simulink model "PackAndSend"  (R2016b)
settings: Solver=FixedStepDiscrete  StartTime=0.0  StopTime=inf  FixedStep=sCoreParams.core.stepPeriod  RelTol=1e-3  EnableMultiTasking=on
values from neighbouring files (symbols this model uses):
  sCoreParams = InitCoreParams    [ClosedLoopStimConsole.m]    (also in CompileModelComplete.m; NeuroModConsole.m)
libraries: simulink x2, xpclib x2
settings Model: Creator=User  LastModifiedBy=rzelmann
settings SolverCC: EnableConcurrentExecution=on
settings DataIOCC: SaveFormat=Array  SaveOutput=off  SignalLogging=off  DSMLogging=off  SaveTime=off
settings OptimizationCC: BlockReduction=off  DefaultParameterBehavior=Inlined  OptimizeBlockIOStorage=off  BufferReuse=off  GlobalBufferReuse=off  ExpressionFolding=off  LocalBlockOutputs=off
settings DebuggingCC: UnderspecifiedInitializationDetection=Classic  MergeDetectMultiDrivingBlocksExec=none  SolverPrmCheckMsg=warning  StateNameClashWarn=warning  SFUnexpectedBacktrackingDiag=warning  SFNoUnconditionalDefaultTransitionDiag=warning  SFExecutionAtInitializationDiag=none
settings HardwareCC: ProdBitPerPointer=32  ProdBitPerSizeT=32  ProdBitPerPtrDiffT=32  ProdLargestAtomicFloat=None  ProdWordSize=32  ProdLongLongMode=on  ProdHWDeviceType=Generic->32-bit x86 compatible
settings ModelReferenceCC: ModelReferenceNumInstancesAllowed=Single  PropagateSignalLabelsOutOfModel=off
settings RTWCC: SystemTargetFile=slrt.tlc  TemplateMakefile=slrt_default_tmf  Description=Simulink Real-Time  RTWCompilerOptimization=on
settings SimulinkRealTimeCC: xPCisModelTimeout=off
settings ConfigComp: CovMetricSettings=dw  CovHtmlReporting=on  CovSaveCumulativeToWorkspaceVar=on  CovSaveSingleToWorkspaceVar=on  CovExternalEMLEnable=off

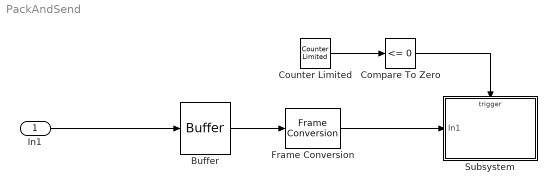
== system PackAndSend ==
  In1 : Inport  PortDimensions=[1 sCoreParams.write.maxSignalsPerStep]  SampleTime=sCoreParams.core.stepPeriod  Interpolate=off
  Buffer : Buffer  N=sCoreParams.write.broadcastSamp  V=sCoreParams.write.broadcastSamp-1  TreatMby1Signals=One channel
  Compare To Zero : simulink/Logic and Bit Operations/Compare To Zero  relop=<=  OutDataTypeStr=boolean
  Counter Limited : simulink/Sources/Counter Limited  uplimit=sCoreParams.write.broadcastSamp-1  tsamp=-1
  Frame Conversion : FrameConversion  InheritSamplingMode=off  OutFrame=Sample-based
  Subsystem : Subsystem
  wires:
  Buffer/1 -> Frame Conversion/1
  Counter Limited/1 -> Compare To Zero/1
  Compare To Zero/1 -> Subsystem/Trigger
  Frame Conversion/1 -> Subsystem/1(In1)
  In1/1 -> Buffer/1

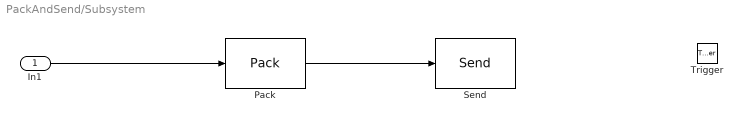
== system PackAndSend/Subsystem ==
  In1 : Inport
  Trigger : TriggerPort  VariantControl=Variant  PortDimensions=1
  Pack : xpclib/UDP/Pack  datatypes={'double'}  byteAlign=1
  Send : xpclib/UDP/Send  ipAddress=255.255.255.255  ipPort=59123  localPort=59121  vblLen=off  sampletime=-1
  wires:
  Pack/1 -> Send/1
  In1/1 -> Pack/1
